simulink model "orbitalTransferSim_v2"  (R2020b)
settings: Solver=FixedStepAuto  StartTime=0.0  StopTime=24*3600*1  FixedStep=0.25  RelTol=1e-12
values from neighbouring files (symbols this model uses):
  IC = [-Xi 0 0        0 -v 0         M]    [main.m]
  ISP = 2100*0.99    (= 2079)    [main.m]
  r_des = 35786+Re    (= 42164.14)    [main.m]
  theta_0 = 24*pi    (= 75.3982236862)    [main.m]
  thrust = 5    [main.m]
settings Model: Creator=mach1337  LastModifiedBy=mach1337

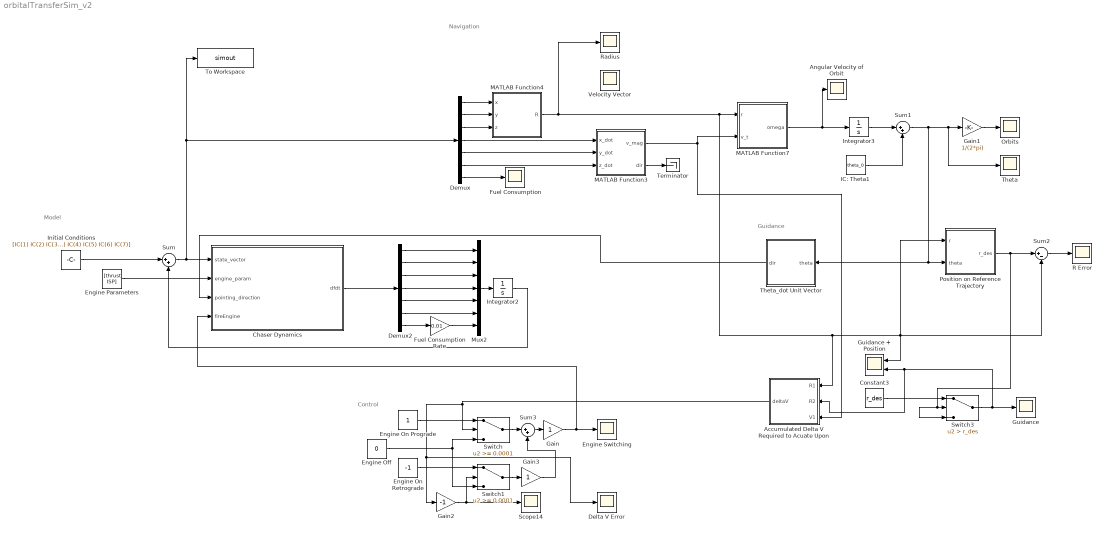
== system orbitalTransferSim_v2 ==
  note: Model
  note: Guidance
  note: Navigation
  note: Control
  Accumulated Delta V Required to Acuate Upon : MATLAB Function  TreatAsAtomicUnit=on
  Angular Velocity of Orbit : Scope
  Chaser Dynamics : MATLAB Function  TreatAsAtomicUnit=on
  Constant3 : Constant  Value=r_des
  Delta V Error : Scope
  Demux : Demux  Outputs=7
  Demux2 : Demux  Outputs=7
  Engine Off : Constant  Value=0  OutDataTypeStr=Inherit: Inherit via back propagation
  Engine On Prograde : Constant
  Engine On Retrograde : Constant  Value=-1
  Engine Parameters : Constant  Value=[thrust ISP]
  Engine Switching : Scope
  Fuel Consumption : Scope
  Fuel Consumption Rate : Gain  Gain=0.01
  Gain : Gain
  Gain1 : Gain  Gain=1/(2*pi)
  Gain2 : Gain  Gain=-1
  Gain3 : Gain
  Guidance : Scope
  Guidance + Position : Scope  NumInputPorts=2
  IC: Theta1 : Constant  Value=theta_0
  Initial Conditions : Constant  Value=[IC(1) IC(2) IC(3) IC(4) IC(5) IC(6) IC(7)]
  Integrator2 : Integrator
  Integrator3 : Integrator
  MATLAB Function3 : MATLAB Function  TreatAsAtomicUnit=on
  MATLAB Function4 : MATLAB Function  TreatAsAtomicUnit=on
  MATLAB Function7 : MATLAB Function  TreatAsAtomicUnit=on
  Mux2 : Mux  Inputs=7
  Orbits : Scope
  Position on Reference Trajectory : MATLAB Function  TreatAsAtomicUnit=on
  R Error : Scope
  Radius : Scope
  Scope14 : Scope
  Sum : Sum  Inputs=|++
  Sum1 : Sum  Inputs=|++
  Sum2 : Sum  Inputs=|+-
  Sum3 : Sum  Inputs=|++
  Switch : Switch  Threshold=0.0001
  Switch1 : Switch  Threshold=0.0001
  Switch3 : Switch  Criteria=u2 > Threshold  Threshold=r_des
  Terminator : Terminator
  Theta : Scope
  Theta_dot Unit Vector : MATLAB Function  TreatAsAtomicUnit=on
  To Workspace : ToWorkspace  VariableName=simout  SaveFormat=Timeseries  SampleTime=-1
  Velocity Vector : Scope
  wires:
  Engine Parameters/1 -> Chaser Dynamics/2(engine_param)
  Initial Conditions/1 -> Sum/1
  Sum/1 -> To Workspace/1, Demux/1, Chaser Dynamics/1(state_vector)
  Demux/4 -> MATLAB Function3/1(x_dot)
  Demux/5 -> MATLAB Function3/2(y_dot)
  Demux/6 -> MATLAB Function3/3(z_dot)
  Demux/7 -> Fuel Consumption/1
  Chaser Dynamics/1(dfdt) -> Demux2/1
  Engine On Prograde/1 -> Switch/1
  Demux2/7 -> Fuel Consumption Rate/1
  Fuel Consumption Rate/1 -> Mux2/7
  Demux2/6 -> Mux2/6
  Demux2/5 -> Mux2/5
  Demux2/4 -> Mux2/4
  Demux2/3 -> Mux2/3
  Demux2/2 -> Mux2/2
  Demux2/1 -> Mux2/1
  Demux/3 -> MATLAB Function4/3(z)
  Demux/2 -> MATLAB Function4/2(y)
  Demux/1 -> MATLAB Function4/1(x)
  MATLAB Function4/1(R) -> MATLAB Function7/1(r), Sum2/2, Guidance + Position/1, Position on Reference Trajectory/1(r), Accumulated Delta V Required to Acuate Upon/1(R1), Radius/1
  Gain/1 -> Chaser Dynamics/4(fireEngine), Engine Switching/1
  Mux2/1 -> Integrator2/1
  Integrator2/1 -> Sum/2
  MATLAB Function3/1(v_mag) -> MATLAB Function7/2(v_t), Accumulated Delta V Required to Acuate Upon/3(V1)
  MATLAB Function7/1(omega) -> Integrator3/1, Angular Velocity of Orbit/1
  IC: Theta1/1 -> Sum1/2
  Integrator3/1 -> Sum1/1
  Sum1/1 -> Theta_dot Unit Vector/1(theta), Position on Reference Trajectory/2(theta), Theta/1, Gain1/1
  Gain1/1 -> Orbits/1
  Position on Reference Trajectory/1(r_des) -> Sum2/1, Switch3/3, Switch3/2
  Sum2/1 -> R Error/1
  Engine Off/1 -> Switch1/3, Switch/3
  Engine On Retrograde/1 -> Switch1/1
  Gain2/1 -> Scope14/1, Switch1/2
  Switch/1 -> Sum3/1
  Sum3/1 -> Gain/1
  Constant3/1 -> Switch3/1
  Switch3/1 -> Guidance + Position/2, Accumulated Delta V Required to Acuate Upon/2(R2), Guidance/1
  Switch1/1 -> Gain3/1
  Gain3/1 -> Sum3/2
  Theta_dot Unit Vector/1(dir) -> Chaser Dynamics/3(pointing_direction)
  MATLAB Function3/2(dir) -> Terminator/1
  Accumulated Delta V Required to Acuate Upon/1(deltaV) -> Delta V Error/1, Gain2/1, Switch/2

== matlab function orbitalTransferSim_v2/Theta_dot Unit Vector ==
  data: dir output; theta input
function dir = fcn(theta)


xDir = sin(theta);
yDir = -cos(theta);
% 
% if x < 0 && y < 0
%     xDir = cos(theta);
% elseif  
%     xDir = cos(theta);    
% end
% 
% if x < 0 && y < 0
%     yDir = -sin(theta);
% elseif  
%     yDir = -sin(theta);    
% end


dir = [xDir yDir 0];

== matlab function orbitalTransferSim_v2/Chaser Dynamics ==
  data: dfdt output; state_vector input; engine_param input; pointing_direction input; fireEngine input
function dfdt = EOM(state_vector, engine_param, pointing_direction, fireEngine)

    % Constants
    mu=3.986005*10^5;         % [km^3/s^2] 
    g0=9.8066;                % [m/s] gravity

    % Engine Parameters
    thrust = engine_param(1); % [N] engine thrust 
    ISP = engine_param(2);    % [s] specific impulse engine

    dfdt = zeros(size(state_vector));
    x     = state_vector(1); % x
    y     = state_vector(2); % y
    z     = state_vector(3); % z
    x_dot = state_vector(4); % dx/dt
    y_dot = state_vector(5); % dy/dt
    z_dot = state_vector(6); % dz/dt
    m     = state_vector(7); % mass
%    theta = state_vector(8);
 
    r=sqrt(x^2+y^2+z^2);

    if fireEngine ~= 0
        vel = [x_dot y_dot z_dot];
        vel_dir = vel/norm(vel);
        pos = [x y z];
        pos_dir = pos/norm(pos);
        F = (thrust/m)/1000;
        F = F.*pointing_direction.*fireEngine;
        %F = F.*pos_dir;
        Fx = F(1);
        Fy = F(2);
        Fz = F(3);
        mass = -thrust/(ISP*g0);
    else
        Fx = 0;
        Fy = 0;
        Fz = 0;
        mass = 0;
    end

    dfdt(1) = x_dot;
    dfdt(2) = y_dot;
    dfdt(3) = z_dot;
    dfdt(4) = -mu*x/r^3 + Fx;
    dfdt(5) = -mu*y/r^3 + Fy;
    dfdt(6) = -mu*z/r^3 + Fz;
    dfdt(7) = mass;

== matlab function orbitalTransferSim_v2/MATLAB Function3 ==
  data: x_dot input; v_mag output; y_dot input; z_dot input; dir output
function [v_mag, dir]= vel(x_dot, y_dot, z_dot)

v = [x_dot, y_dot, z_dot];

dir = v/norm(v);
v_mag = sqrt(x_dot^2 + y_dot^2 + z_dot^2);

== matlab function orbitalTransferSim_v2/MATLAB Function4 ==
  data: x input; R output; y input; z input
function R = fcn(x, y, z)

R = sqrt(x^2 + y^2 + z^2);

== matlab function orbitalTransferSim_v2/MATLAB Function7 ==
  data: r input; omega output; v_t input
function omega = fcn(r, v_t)

omega = v_t/r;

== matlab function orbitalTransferSim_v2/Position on Reference Trajectory ==
  data: r input; r_des output; theta input
function r_des = fcn(r, theta)

a = -0.2;
n = 0.40345;
r_des = abs(a.*theta.^(1./n));

== matlab function orbitalTransferSim_v2/Accumulated Delta V Required to Acuate Upon ==
  data: R1 input; R2 input; deltaV output; V1 input
function deltaV = fcn(R1, R2, V1)

a = (R1 + R2)/2;

mu = 3.9860e+05;

%V2B = sqrt(mu/R1)*(sqrt(2*R2/(R1+R2)) - 1)+V1;
%V2B = sqrt(mu/R1)*(sqrt(2*R2/(R1+R2)) - 1);

deltaV = sqrt(mu*( 2/R1 - 1/a ))-V1;
